simulink model "Braking_technique_DC_Dynamic_Braking"  (R2021b)
settings: Solver=VariableStepAuto  StartTime=0.0  StopTime=5  RelTol=1e-3  EnableMultiTasking=on
libraries: spsBreakerLib x2, spsDCVoltageSourceLib x2, spsSeriesRLCBranchLib x1, spsDCMachineLib x1, spspowerguiLib x1
settings Model: Creator=Mostafa  LastModifiedBy=Unicorn
settings SolverCC: AlgebraicLoopSolver=TrustRegion
settings DataIOCC: ReturnWorkspaceOutputs=off
settings OptimizationCC: LifeSpan=inf
settings DebuggingCC: SFUnexpectedBacktrackingDiag=warning  SFNoUnconditionalDefaultTransitionDiag=warning  SFMachineParentedDataDiag=warning  ArithmeticOperatorsInVariantConditions=warning
settings SFSimCC: SimUseLocalCustomCode=off  CustomCodeUndefinedFunction=UseInterfaceOnly
settings RTWCC: RTWUseLocalCustomCode=off
settings CodeAppCC: StateflowObjectComments=on
settings GRTTargetCC: TargetLangStandard=C89/C90 (ANSI)
settings ConfigComp: CovMetricSettings=dw  CovSaveCumulativeToWorkspaceVar=on  CovSaveSingleToWorkspaceVar=on  CovExternalEMLEnable=off
settings SimscapeCC: SimscapeNormalizeSystem=off

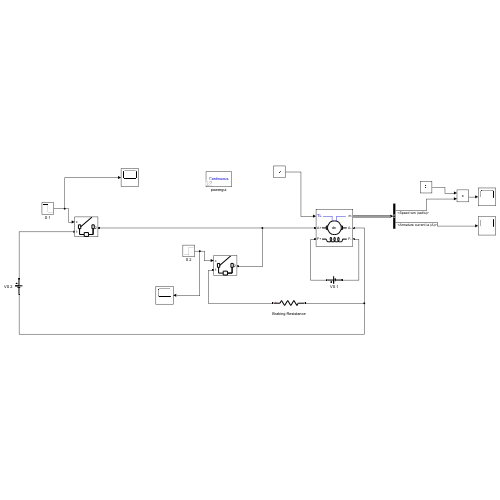
[thumbnail: Simulink's stored preview of the top-level diagram]
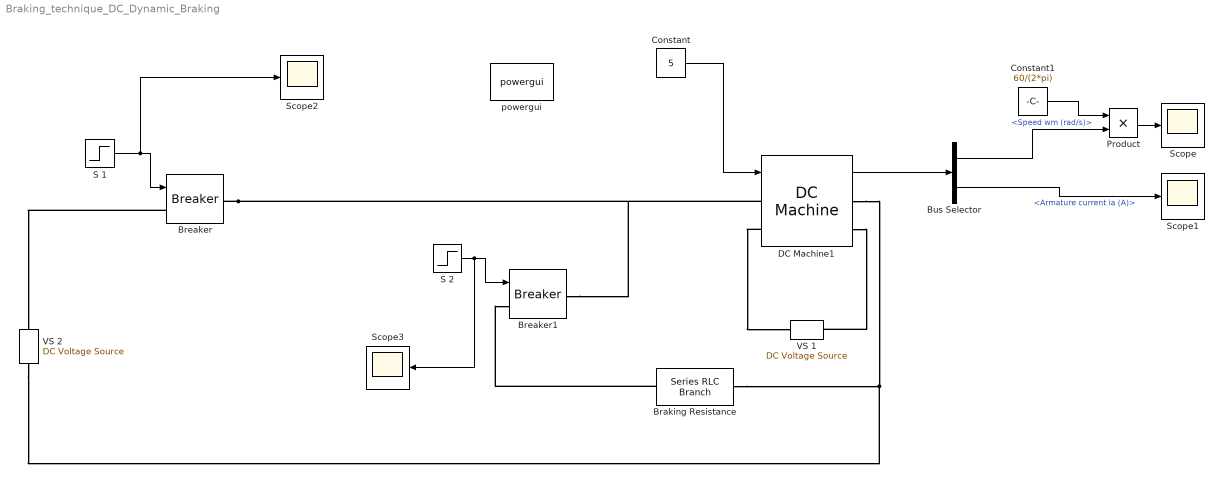
== system Braking_technique_DC_Dynamic_Braking ==
  Braking Resistance : spsSeriesRLCBranchLib/Series RLC Branch  LConnTagsString=__new0  RConnTagsString=__new0  BranchType=R  Resistance=2  Inductance=1e-3  SetiL0=off  InitialCurrent=0  Capacitance=1e-6  Setx0=off  InitialVoltage=0  Measurements=None
  Breaker : spsBreakerLib/Breaker  InitialState=0  SwitchingTimes="[1/60  5/60]"  External=on  BreakerResistance=0.01  SnubberResistance=1e6  SnubberCapacitance=inf  Measurements=None  MoreParameters=on  NoBreakLoop=off
      settings: SourceProductBaseCode=PS
  Breaker1 : spsBreakerLib/Breaker  InitialState=0  SwitchingTimes="[1/60  5/60]"  External=on  BreakerResistance=0.01  SnubberResistance=1e6  SnubberCapacitance=inf  Measurements=None  MoreParameters=on  NoBreakLoop=off
      settings: SourceProductBaseCode=PS
  Bus Selector : BusSelector  OutputSignals=Speed wm (rad/s),Armature current ia (A)
  Constant : Constant  Value=5
  Constant1 : Constant  Value=60/(2*pi)
  DC Machine1 : spsDCMachineLib/DC Machine  PresetModel=No  MechanicalLoad=Torque TL  FieldType=Wound  ShowDetailedParameters=on  MeasurementBus=off  RLa="[ 0.5  0.012]"  RLf="[ 110  120]"  Laf=1.8  MachineConstant=Torque constant (N.m/A)  Ke=1.8  Kt=1.8  J=0.5  Bm=0  Tf=0  w0=1  Ifinit=1  TsPowergui=0  TsBlock=-1
  Product : Product
  S 1 : Step  Time=0.5296  Before=1  After=0  SampleTime=0
  S 2 : Step  Time=0.5296  SampleTime=0
  Scope{,1..3} (4 alike) : Scope
  VS 1 : spsDCVoltageSourceLib/DC Voltage Source  Amplitude=110  Measurements=None
  VS 2 : spsDCVoltageSourceLib/DC Voltage Source  Amplitude=220  Measurements=None
  powergui : spspowerguiLib/powergui  Priority=1  SimulationMode=Continuous  SampleTime=50e-6  frequency=60  Iterations=50  frequencyindice=0  Pbase=100e6  ErrMax=1e-4  UnitsV=kV  UnitsW=MW  buscounter=0  FunctionMessages=off  echomessages=off  EnableUseOfTLC=off  CurrentSourceSwitches=on  DisableSnubberDevices=off  DisableRonSwitches=off  DisableVfSwitches=off  DisplayEquations=off  AutomaticDiscreteSolvers=off  SolverType=Tustin/Backward Euler (TBE)  Interpol=off  ExternalGateDelay=off  methode=off  Ts=10  x0status=blocks  SPID=off  SwTol=0  HookPort=off  NonlinearTolerance=1e-4  nMaxIteration=100  ContinueOnMaxIteration=off  RestoreLinks=warning  ResistiveCurrentMeasurement=off  Frange=[0:2:500]  Ylog=off  Xlog=on  ShowGrid=off  save=off  variable=ZData  structure=0  ZoomFFT=off  StartTime=0.0  cycles=1  DisplayStyle=1  fundamental=60  FreqAxis=off  MaxFrequency=1000  frequencyindicesteady=1  RmsSteady=1  display=off
  wires:
  Constant/1 -> DC Machine1/1
  DC Machine1/1 -> Bus Selector/1
  S 1/1 -> Scope2/1, Breaker/1
  S 2/1 -> Scope3/1, Breaker1/1
  Bus Selector/2 -> Scope1/1  "<Armature current ia (A)>"
  Product/1 -> Scope/1
  Constant1/1 -> Product/1
  Bus Selector/1 -> Product/2  "<Speed wm (rad/s)>"
  connections:
  VS 2/LConn1 -- DC Machine1/RConn1 -- Braking Resistance/RConn1
  DC Machine1/RConn2 -- VS 1/LConn1
  DC Machine1/LConn2 -- VS 1/RConn1
  Breaker/RConn1 -- DC Machine1/LConn1 -- Breaker1/RConn1
  Breaker/LConn1 -- VS 2/RConn1
  Braking Resistance/LConn1 -- Breaker1/LConn1
